simulink model "Noa_Nofusion_angle"  (R2020b)
settings: Solver=FixedStepDiscrete  StartTime=0.0  StopTime=Inf  FixedStep=0.01  RelTol=1e-3
PostLoadFcn:
  | if any(exist('dsrtsu_mdlpostloadfcn', 'file') ~= 0), dsrtsu_mdlpostloadfcn('Execute', bdroot); end
InitFcn:
  | , if any(exist('rtifpga_mdlclblib', 'file') ~= 0), rtifpga_mdlclblib('Init', bdroot); end,
  | , if any(exist('dsmpb_private', 'file') ~= 0), dsmpb_private('dsmpb_mdlclblib', 'Init', bdroot); end,
undefined symbols (not defined in the file): ACC_TimeGap_DecSetSwt, ACC_TimeGap_IncSetSwt, AccelPedalPosn, AccelPedalPosnVldty, AccelPedlPosnDiagc, AccPedalOverride, ACU_ShiftInProgress, ADAS_Posn_CurLane, AESSwtReq, ALC_SwtReq, BrkPedalSts, CC_ACC_CANCEL_OFFSwt, CC_ACC_CRUISE_OFFSwt, CC_ACC_DecSetSpd_SetSwt, CC_ACC_IncSetSpd_ResuSwt, CC_ACCSwtErr, CharSpd_ms, CSA_NODE, CURRENT_GEAR, CurrentGearValid, DiscIntNeverNeededParam, DrvDoorSts, DrvSBR, DrvTrqReqOvld, ECMACCInterface, ECMRespACC, ELKSwtReq, EngLimpHomeSts, EngSpd, EngState, EngState_PHEV, EngTrqMaxActSpd, EngTrqMinAct, EPS_DrvInpTrqVal_HighReslolution, EPS_FailSts, EPS_LKATorqOvrlDlvd, EPS_LKATorqOvrlDlvdVld, EPS_LKATrqOvlDlvdSts, EPS_SteerMod, EPS_TrqSnsrSts, EQ4_APPINFO, EQ4_LA_ELEM, EQ4_LA_HDR, EQ4_LAP_ELEM, EQ4_LAP_HDR, EQ4_LH_ELEM, EQ4_LH_HDR, EQ4_LRE_ELEM, EQ4_LRE_HDR, ESS_PedSwtReq, ESS_VehSwtReq, FFogLmpSts_F_Pbox, FLWheelDriveDirection, FLWheelSpd, FrntWiprSwtSts, FrntWshrSwtSts, FRWheelDriveDirection, FRWheelSpd, HazardLmpSwtSts, HCU_AccelPedalPosn_Diag ... (+151)
libraries: simulink x138, dsmpblib x33, canfdmsglib x10
(part 14 of 17)

== matlab function Noa_Nofusion_angle/TOS2/Subsystem1/ACCOSM/HWA_Task100ms1/Trajectory/Trajectory/AssignHighPriorityObjects ==
  data: ObjNumber input; TrajNumber input; BufNumber input; SlipDisLim input; ObjPrio input; ObjMatrix input; VxvRef input; ObjCntAlive input; ObjClass input; ObjDxv input; ObjDyv input; TrajUsedK1 input; TrajHistBufferBTrajEndK1 input; ObjTrajNumberK1 input; TrajCurrentIndexK1 input; TrajHistBufferBValidK1 input; TrajHistBufferDxvK1 input; TrajHistBufferDyvK1 input; TrajHistBufferTTimeStampK1 input; TrajHistBufferClassK1 input; TrajUsed output boolean; TrajHistBufferBTrajEnd output boolean; ObjTrajNumber output uint8; TrajCurrentIndex output uint8; TrajHistBufferBValid output boolean; TrajHistBufferDxv output single; TrajHistBufferDyv output single; TrajHistBufferTTimeStamp output single; TrajHistBufferClass output uint8
function [TrajUsed,TrajHistBufferBTrajEnd,ObjTrajNumber,TrajCurrentIndex,TrajHistBufferBValid,...
    TrajHistBufferDxv,TrajHistBufferDyv,...
    TrajHistBufferTTimeStamp,TrajHistBufferClass] = fcn(...
    ObjNumber,TrajNumber,BufNumber,SlipDisLim,ObjPrio,ObjMatrix,VxvRef,ObjCntAlive,ObjClass,ObjDxv,ObjDyv,...
    TrajUsedK1,TrajHistBufferBTrajEndK1,ObjTrajNumberK1,TrajCurrentIndexK1,...
    TrajHistBufferBValidK1,TrajHistBufferDxvK1,TrajHistBufferDyvK1,...
    TrajHistBufferTTimeStampK1,TrajHistBufferClassK1)

[TrajUsed,TrajHistBufferBTrajEnd,ObjTrajNumber,TrajCurrentIndex,TrajHistBufferBValid,...
    TrajHistBufferDxv,TrajHistBufferDyv,...
    TrajHistBufferTTimeStamp,TrajHistBufferClass] = Traj_AssignHighPriorityObjects(...
    ObjNumber,TrajNumber,BufNumber,SlipDisLim,ObjPrio,ObjMatrix,VxvRef,ObjCntAlive,ObjClass,ObjDxv,ObjDyv,...
    TrajUsedK1,TrajHistBufferBTrajEndK1,ObjTrajNumberK1,TrajCurrentIndexK1,...
    TrajHistBufferBValidK1,TrajHistBufferDxvK1,TrajHistBufferDyvK1,...
    TrajHistBufferTTimeStampK1,TrajHistBufferClassK1);
end

== matlab function Noa_Nofusion_angle/TOS2/Subsystem1/ACCOSM/HWA_Task100ms1/Trajectory/Trajectory/CalcCompensateEgoVehMove ==
  data: BufNumber input; TrajNumber input; tCycle input; dDeltaX input; dDeltaY input; CosOfPsi input; SinOfPsi input; TrajHistBufferBValidK1 input; TrajHistBufferDxvK1 input; TrajHistBufferDyvK1 input; TrajHistBufferBValid output; TrajHistBufferDxv output; TrajHistBufferDyv output; TrajHistBufferTTimeStampK1 input; TrajHistBufferTTimeStamp output
function [TrajHistBufferBValid,TrajHistBufferDxv,TrajHistBufferDyv,...
    TrajHistBufferTTimeStamp] = ...
    Compensate(BufNumber,TrajNumber,tCycle,dDeltaX,dDeltaY,CosOfPsi,SinOfPsi,...
    TrajHistBufferBValidK1,TrajHistBufferDxvK1,TrajHistBufferDyvK1,...
    TrajHistBufferTTimeStampK1)
%#codegen
TrajHistBufferBValid = TrajHistBufferBValidK1;
TrajHistBufferDxv = TrajHistBufferDxvK1;
TrajHistBufferDyv = TrajHistBufferDyvK1;
TrajHistBufferTTimeStamp = TrajHistBufferTTimeStampK1;

for i=1:TrajNumber
    for j=1:BufNumber
        if TrajHistBufferBValid(i,j)==true
            t_dx = TrajHistBufferDxv(i,j)-dDeltaX;
            t_dy = TrajHistBufferDyv(i,j)-dDeltaY;
            t_dxTmp = t_dx*CosOfPsi+t_dy*SinOfPsi;
            t_dyTmp = -t_dx*SinOfPsi+t_dy*CosOfPsi;
            if (t_dxTmp>-255)&&(t_dxTmp<255)&&(t_dyTmp>-255)&&(t_dyTmp<255)
                TrajHistBufferDxv(i,j) = t_dxTmp;
                TrajHistBufferDyv(i,j) = t_dyTmp;
            else
                TrajHistBufferBValid(i,j) = false;
            end
            
            TrajHistBufferTTimeStamp(i,j) = min(TrajHistBufferTTimeStamp(i,j)+tCycle,32);
            
            if TrajHistBufferDxv(i,j)<-1
                TrajHistBufferBValid(i,j) = false;
            end
        end
    end
end

== matlab function Noa_Nofusion_angle/TOS2/Subsystem1/ACCOSM/HWA_Task100ms1/Trajectory/Trajectory/CalcEgoVehMove ==
  data: dDeltaX output single size=1; tCycle input size=1; Kap input size=1; Vego input size=1; alpSideSlipAngle input size=1; dDeltaY output single size=1; CosOfPsi output single size=1; SinOfPsi output single size=1; WheelTrack input; SlipDislim output; Vch input
function [dDeltaX,dDeltaY,CosOfPsi,SinOfPsi,SlipDislim] = EgoVehicleMovement(tCycle,Kap,Vego,alpSideSlipAngle,WheelTrack,Vch)
%#codegen
if Kap==0
    dDeltaX = Vego*tCycle;
    dDeltaY = single(0);
    CosOfPsi = single(1);
    SinOfPsi = single(0);
    SlipDislim = Vch*1000;
else
    SlipDislim = max(WheelTrack*1000,min(tCycle*Vego,Kap*15));
    t_Psi = Kap*Vego*tCycle;
    SinOfPsi = sin(t_Psi);
    CosOfPsi = cos(t_Psi);
    t_dDeltaXTemp = SinOfPsi/Kap;
    t_dDeltaYTemp = 2*(sin(t_Psi/2)*sin(t_Psi/2))/Kap;
    dDeltaX = min(cos(alpSideSlipAngle)*t_dDeltaXTemp - sin(alpSideSlipAngle)*t_dDeltaYTemp,SlipDislim);
    dDeltaY = sin(alpSideSlipAngle)*t_dDeltaXTemp + cos(alpSideSlipAngle)*t_dDeltaYTemp;
end

== matlab function Noa_Nofusion_angle/TOS2/Subsystem1/ACCOSM/HWA_Task100ms1/Trajectory/Trajectory/Priority ==
  data: ObjNumber input; ObjValid input; ObjPrio output single; ObjClass input; ObjDx input; ObjMatrix output single
function [ObjPrio,ObjMatrix] = fcn(ObjNumber,ObjValid,ObjClass,ObjDx)
%#codegen
ObjPrio = single(zeros(15,1));

for i=1:ObjNumber
    if ObjValid(i)
        if ObjDx(i)<0
            ObjPrio(i)=single(0);
        else
            if (ObjClass(i)==2)||(ObjClass(i)==3)||(ObjClass(i)==5)
                t_ObjPrio=single(2*255);
            else
                t_ObjPrio=single(255);
            end
            ObjPrio(i) = t_ObjPrio - ObjDx(i);
        end
    else
        ObjPrio(i)=single(0);
    end
end

ObjMatrix=ObjPrio;

t_h=1;
while 1
    t_h = t_h*3+1;
    if t_h>=ObjNumber
        break;
    end
end

%   t_h = 121;
while 1
    t_h = fix(t_h/3);
    for i=(t_h+1):ObjNumber
        j=i;
        t_zw=ObjMatrix(i);
        while (j>t_h)&&(t_zw<ObjMatrix(j-t_h))
            ObjMatrix(j)=ObjMatrix(j-t_h);
            j=j-t_h;
        end
        ObjMatrix(j)=t_zw;
    end
    if t_h==1
        break;
    end
end

== matlab function Noa_Nofusion_angle/TOS2/Subsystem1/ACCOSM/HWA_Task100ms1/Trajectory/Trajectory/ReleaseLowPriorityObjects ==
  data: TrajUsed output; ObjNumber input; TrajNumber input; ObjPrio input; ObjMatrix input; ObjValid input; TrajCurrentIndex input; TrajUsedK1 input; TrajHistBufferBTrajEndK1 input; ObjTrajNumberK1 input; TrajHistBufferBTrajEnd output; ObjTrajNumber output
function [TrajUsed,TrajHistBufferBTrajEnd,ObjTrajNumber] =...
    fcn(ObjNumber,TrajNumber,ObjPrio,ObjMatrix,ObjValid,TrajCurrentIndex,...
    TrajUsedK1,TrajHistBufferBTrajEndK1,ObjTrajNumberK1)
%#codegen
TrajHistBufferBTrajEnd = TrajHistBufferBTrajEndK1;
TrajUsed = TrajUsedK1;
ObjTrajNumber = ObjTrajNumberK1;
ObjPrioLimit = ObjMatrix(ObjNumber-TrajNumber);

for i=1:ObjNumber
    if ObjValid(i)
        if (ObjPrio(i)==0)||(ObjPrio(i)<=ObjPrioLimit)
            j = ObjTrajNumber(i);
            if j<(TrajNumber+1)
                t = TrajCurrentIndex(j);
                TrajHistBufferBTrajEnd(j,t)=1;
                TrajUsed(j)=0;
                ObjTrajNumber(i)=255;
            end
        end
    end
end

== matlab function Noa_Nofusion_angle/TOS2/Subsystem1/ACCOSM/HWA_Task100ms1/Trajectory/Trajectory/StoreEgoTrajectory ==
  data: Pa output single; Pb output single; Pc output single; Pd output single; BufNumber input; tCycle input; EgoTrajHistCurrentIndex output uint8; EgoDDeltaX input; EgoDDeltaY input; EgoCosOfPsi input; EgoSinOfPsi input; EgoTrajHistDxv output; EgoTrajHistDyv output; EgoTrajHistTTimeStamp output; EgoTrajHistCurrentIndexK1 input; EgoTrajHistDxvK1 input single; EgoTrajHistDyvK1 input single; EgoTrajHistTTimeStampK1 input single
function [Pa,Pb,Pc,Pd,EgoTrajHistCurrentIndex,EgoTrajHistDxv,EgoTrajHistDyv,EgoTrajHistTTimeStamp]...
    = fcn(BufNumber,tCycle,EgoDDeltaX,EgoDDeltaY,EgoCosOfPsi,EgoSinOfPsi,...
    EgoTrajHistCurrentIndexK1,EgoTrajHistDxvK1,EgoTrajHistDyvK1,EgoTrajHistTTimeStampK1)
%#codegen
EgoTrajHistCurrentIndex = EgoTrajHistCurrentIndexK1;
EgoTrajHistDxv = EgoTrajHistDxvK1;
EgoTrajHistDyv = EgoTrajHistDyvK1;
EgoTrajHistTTimeStamp = EgoTrajHistTTimeStampK1;
% alpWheelAngleOffset = alpWheelAngleOffsetK1;

t_IdxActualElement = EgoTrajHistCurrentIndex;
if t_IdxActualElement==BufNumber
    t_IdxNextElement=uint8(1);
else
    t_IdxNextElement=t_IdxActualElement+1;
end

Temp1 = EgoTrajHistDxv(t_IdxActualElement) - EgoDDeltaX;
Temp2 = EgoTrajHistDyv(t_IdxActualElement) - EgoDDeltaY;
dDeltaS = Temp1*Temp1 + Temp2*Temp2;
t_AddPosition = ((EgoTrajHistTTimeStamp(t_IdxActualElement)+tCycle)>0.3);
t_AddPosition = t_AddPosition&(dDeltaS>4);
t_AddPosition = t_AddPosition|(dDeltaS>100);
for iBuf=1:BufNumber
    if (t_AddPosition==1)&&(iBuf==t_IdxNextElement)
        EgoTrajHistDxv(iBuf)=single(0);
        EgoTrajHistDyv(iBuf)=single(0);
        EgoTrajHistTTimeStamp(iBuf)=single(0);
        EgoTrajHistCurrentIndex = t_IdxNextElement;
    else
        dX = EgoTrajHistDxv(iBuf)-EgoDDeltaX;
        dY = EgoTrajHistDyv(iBuf)-EgoDDeltaY;
        if (EgoTrajHistDxv(iBuf)>-255)&&(dX>-255)&&(dX<255)&&(dY>-255)&&(dY<255)
            Temp1 = dX*EgoCosOfPsi + dY*EgoSinOfPsi;
            Temp2 = -dX*EgoSinOfPsi + dY*EgoCosOfPsi;
            if (Temp1>-255)&&(Temp1<255)&&(Temp2>-255)&&(Temp2<255)
                EgoTrajHistDxv(iBuf)=Temp1;
                EgoTrajHistDyv(iBuf)=Temp2;
                tDt = EgoTrajHistTTimeStamp(iBuf)+tCycle;
                if tDt>32
                    tDt=single(32);
                end
                EgoTrajHistTTimeStamp(iBuf) = tDt;
            else
                EgoTrajHistDxv(iBuf)=single(-255);
                EgoTrajHistDyv(iBuf)=single(-255);
                EgoTrajHistTTimeStamp(iBuf) = single(32);
            end
        else
            EgoTrajHistDxv(iBuf)=single(-255);
            EgoTrajHistDyv(iBuf)=single(-255);
            EgoTrajHistTTimeStamp(iBuf) = single(32);
        end
    end
end

t_Index = EgoTrajHistCurrentIndex;
t_Index1 = BufNumber + uint8(23);
t_Index2 = BufNumber + uint8(21);
t_Index3 = BufNumber + uint8(19);

if t_Index1>24
    t_Index1 = t_Index1 - uint8(24);
end
if t_Index2>24
    t_Index2 = t_Index2 - uint8(24);
end
if t_Index3>24
    t_Index3 = t_Index3 - uint8(24);
end

XiMa = [EgoTrajHistDxv(t_Index);EgoTrajHistDxv(t_Index1);EgoTrajHistDxv(t_Index2);EgoTrajHistDxv(t_Index3)];
YiMa = [EgoTrajHistDyv(t_Index);EgoTrajHistDyv(t_Index1);EgoTrajHistDyv(t_Index2);EgoTrajHistDyv(t_Index3)];

[Pa,Pb,Pc,Pd] = pl(XiMa,YiMa);

% if (abs(EgoTrajHistDyv(t_Index1))<0.1)&&(abs(EgoTrajHistDyv(t_Index2))<0.1)&&(abs(EgoTrajHistDyv(t_Index3))<0.1)
%     kapRef = 3*Pa*EgoTrajHistDxv(t_Index2) + 2*Pb;
%     AckConst = min((1+VxvRef*VxvRef/(26*26))*2.68/max(VxvRef,1),32767);
%     alpWheelAngleRef = VxvRef*kapRef*AckConst;
%     Raw = alpWheelAngleMean - alpWheelAngleRef;
%     if VxvRef>7.3
%         alpWheelAngleOffset = (Raw - alpWheelAngleOffset)/10000 + alpWheelAngleOffset;
%     end
% else
%     alpWheelAngleRef = single(255);
% end

== matlab function Noa_Nofusion_angle/TOS2/Subsystem1/ACCOSM/HWA_Task100ms1/VycCalc ==
  data: ObjVyc output single size=15; dxC0 input; aP0 input; bP0 input; aP1 input; bP1 input; ObjValid input boolean size=15; ObjDx input single size=15; ObjVxG input single size=15; ObjVyG input single size=15; ObjYawAngle output
function [ObjVyc,ObjYawAngle] = VycCalc(dxC0,aP0,bP0,aP1,bP1,ObjValid,ObjDx,ObjVxG,ObjVyG)

ObjVyc = single(zeros(15,1));
ObjYawAngle = single(zeros(15,1));

for i=1:15
    if ObjValid(i)
       t_dxv = ObjDx(i);
       t_VxG = ObjVxG(i);
       t_VyG = ObjVyG(i);
       
       if abs(t_VxG)<0.1
          if t_VyG>0.5
              ObjYawAngle(i) = single(1.57);
          end
          if t_VyG<-0.5
              ObjYawAngle(i) = single(-1.57);
          end
       else
           if t_VxG>0
               ObjYawAngle(i) = atan(t_VyG/t_VxG);
           else
               if t_VyG>0
                  ObjYawAngle(i) = single(3.1416) + atan(t_VyG/t_VxG);
               else
                  ObjYawAngle(i) = -single(3.1416) + atan(t_VyG/t_VxG);
               end
           end
       end
       
       t_bParabolaYNLane = single(1);
       if t_dxv<dxC0
          temp1 =  2*aP0*t_dxv + bP0;
          t_bParabolaXNLane = -temp1;
       else
          temp1 =  2*aP1*t_dxv + bP1;
          t_bParabolaXNLane = -temp1;
       end
       t_bParabolaMag = mag(t_bParabolaXNLane,t_bParabolaYNLane);
       t_bParabolaXNLane = t_bParabolaXNLane/t_bParabolaMag;
       t_bParabolaYNLane = t_bParabolaYNLane/t_bParabolaMag;
       temp1 = t_VxG*t_bParabolaXNLane;
       temp2 = t_VyG*t_bParabolaYNLane;
       
       ObjVyc(i) = temp1 + temp2;
    else
       ObjVyc(i) = single(0);
    end
end
end

function out = mag(x,y)
M = max(abs(x),abs(y));
N = min(abs(x),abs(y));
out = M + 0.322*N;
end

== matlab function Noa_Nofusion_angle/TOS2/Subsystem1/ACCOSM/HWA_Task100ms1/dyLaneWidthSteerAdapt ==
  data: kap input; dyLaneAdaptLeft output; dyAdapt input; dyLaneAdaptRight output
function [dyLaneAdaptLeft,dyLaneAdaptRight] = fcn(kap,dyAdapt)

dyLaneAdaptLeft = single(0);
dyLaneAdaptRight = single(0);
if kap>0
    dyLaneAdaptRight = dyAdapt;
end
if kap<0
    dyLaneAdaptLeft = dyAdapt;
end

== matlab function Noa_Nofusion_angle/TOS2/Subsystem1/ACCOSM/HWA_Task100ms1/wCutInVy ==
  data: DycASI output single; ObjValid input boolean size=15; ObjDycCutIn input single size=15; ObjWidth input single size=15; ObjVyc input single size=15; ObjDx input single size=15; ObjDy input single size=15; ObjCnt input uint8 size=15; ObjDycFilt input single size=15; ObjwCutInVyK1 input single size=15; ObjtPrediction4CutIn output single size=15; ObjDycCutInPredict output single size=15; ObjCutIn_b output boolean size=15; ObjwCutInVy output single size=15
function [DycASI,ObjtPrediction4CutIn,ObjDycCutInPredict,ObjCutIn_b,ObjwCutInVy] = ...
    CalcWCutInVy(ObjValid,ObjDycCutIn,ObjWidth,ObjVyc,ObjDx,ObjDy,ObjCnt,...
    ObjDycFilt,ObjwCutInVyK1)
 
ObjwCutInVy = single(zeros(15,1));
ObjtPrediction4CutIn = single(zeros(15,1));
ObjDycCutInPredict = single(zeros(15,1));
DycASI = single(zeros(15,1));
ObjCutIn_b = false(15,1);
 
for i=1:15
    if ObjValid(i)
        dWidth = ObjWidth(i);
        dycASI = ObjDycCutIn(i);
        vyc = ObjVyc(i);
        dx = ObjDx(i);
        dy = ObjDy(i);
        dycFilt = ObjDycFilt(i);
        wCutInVyK1 = ObjwCutInVyK1(i);
  
        temp1 = dycFilt - dycASI;
        if ((dycASI>0)&&(temp1>0.2))||((dycASI<0)&&(temp1<-0.2))
            tauVy = single(1.6);
        else
            tauVy = single(0);
        end
        tauVy = interpolate(single(40),tauVy,single(70),single(0),dx);
        ObjtPrediction4CutIn(i) = tauVy;
        temp1 = vyc*tauVy;
        temp2 = dycASI + temp1;
        
        if (dycASI>0)&&(temp2<0)
            temp2 = single(0);
        else
            if (dycASI<0)&&(temp2>0)
                temp2 = single(0);
            else
                if dycASI==0
                    temp2 = single(0);
                end
            end
        end
        ObjDycCutInPredict(i) = temp2;
        if dycASI>0
            temp1 = temp2 - 0.5*dWidth;
            t_dycASI = max(temp1,single(0));
        else
            temp1 = temp2 + 0.5*dWidth;
            t_dycASI = min(temp1,single(0));
        end
        temp1 = abs(t_dycASI);
        t_wCutInVy = interpolate(single(0),single(1),single(0.7),single(0),temp1);
        if tauVy==0
            t_wCutInVy = single(0);
        end
        
        if dx>0
            fak = abs(dy)/dx; 
        else
            fak = single(0);
        end
        if (ObjCnt(i)<2)||(abs(dy)>=2.4)||(fak>0.25)
           t_wCutInVy = single(0);
        end
       
        temp1 = t_wCutInVy - wCutInVyK1;
        temp1_ub = abs(temp1);
        temp2 = 0.2*temp1_ub;
        if temp1>0
            t_wCutInVy = wCutInVyK1 + temp2;
        else
            t_wCutInVy = wCutInVyK1 - temp2;
        end
        ObjwCutInVy(i) = t_wCutInVy;
        DycASI(i) = t_dycASI;
        if t_wCutInVy>0.7
            ObjCutIn_b(i) = true;
        end
    end
end
end
 
% function out = interpolate(x1,z1,x2,z2,Raw)
% if Raw<=x1
%     out = z1;
% else
%     if Raw>=x2
%         out = z2;
%     else
%         out = z1 + (Raw-x1)*(z2-z1)/(x2-x1);
%     end
% end
% end

== matlab function Noa_Nofusion_angle/TOS2/Subsystem1/ACCOSM/HWA_Task100ms1/wCutOutVy ==
  data: vRef input single size=1; kap input single size=1; tDirIndLeft input single size=1; tDirIndRight input single size=1; ObjValid input boolean size=15; ObjDycCutIn input single size=15; ObjWidth input single size=15; ObjtPrediction4CutOut output single size=15; ObjDycCutOutPredict output single size=15; ObjwCutOutTurnOff output single size=15; ObjVyc input single size=15; ObjDx input single size=15; ObjDy input single size=15; ObjVx input single size=15; ObjVy input single size=15; ObjDyc input single size=15; ObjDrive_b input boolean size=15; ObjCnt input uint8 size=15; ObjDycFilt input single size=15; ObjwCutoutVyK1 input single size=15; ObjwCutoutVy output single size=15
function [ObjtPrediction4CutOut,ObjDycCutOutPredict,ObjwCutOutTurnOff,ObjwCutoutVy] = ...
    CalcWCutOutVy(vRef,kap,tDirIndLeft,tDirIndRight,ObjValid,ObjDycCutIn,ObjWidth,...
    ObjVyc,ObjDx,ObjDy,ObjVx,ObjVy,ObjDyc,ObjDrive_b,ObjCnt,...
    ObjDycFilt,ObjwCutoutVyK1)
 
ObjwCutoutVy = single(zeros(15,1));
ObjtPrediction4CutOut = single(zeros(15,1));
ObjDycCutOutPredict = single(zeros(15,1));
ObjwCutOutTurnOff = single(zeros(15,1));
 
for i=1:15
    if ObjValid(i)
        dWidth = ObjWidth(i);
        dycASI = ObjDycCutIn(i);
        vyc = ObjVyc(i);
        dx = ObjDx(i);
        dy = ObjDy(i);
        vx = ObjVx(i);
        vy = ObjVy(i);
        dyc = ObjDyc(i);
        dycFilt = ObjDycFilt(i);
        wCutoutVyK1 = ObjwCutoutVyK1(i);
        Move_b = ObjDrive_b(i);
        Cnt = ObjCnt(i);
        t_vxTO = vRef + vx;
        t_vxvThreshold = 0.5 - vRef;
        
        temp1 = dycASI - dycFilt;
        if ((dycASI>0)&&(temp1>0.2))||((dycASI<0)&&(temp1<-0.2))
            tauVy = single(1);
        else
            tauVy = single(0);
        end
        tauVy = interpolate(single(40),tauVy,single(70),single(0),dx);
        ObjtPrediction4CutOut(i) = tauVy;
        temp1 = vyc*tauVy;
        temp2 = dycASI + temp1;
        
        if (dycASI>0)&&(temp2<0)
            temp2 = single(0);
        else
            if (dycASI<0)&&(temp2>0)
                temp2 = single(0);
            else
                if dycASI==0
                    temp2 = single(0);
                end
            end
        end
        ObjDycCutOutPredict(i) = temp2;
        if dycASI>0
            temp1 = temp2 + 0.5*dWidth;
            t_dycASI = max(temp1,single(0));
        else
            temp1 = temp2 - 0.5*dWidth;
            t_dycASI = min(temp1,single(0));
        end
        temp1 = abs(t_dycASI);
        t_wCutoutVy = interpolate(single(0),single(0),single(0.7),single(1),temp1);
        if tauVy==0
            t_wCutoutVy = single(0);
        end
        
        temp1 = t_wCutoutVy - wCutoutVyK1;
        temp1_ub = abs(temp1);
        temp2 = 0.2*temp1_ub;
        if temp1>0
            t_wCutoutVy = wCutoutVyK1 + temp2;
        else
            t_wCutoutVy = wCutoutVyK1 - temp2;
        end
        ObjwCutoutVy(i) = t_wCutoutVy;
        if (dx<30)&&(Move_b==true)&&(vRef>0.5)&&(t_vxTO<6)&&(vx>t_vxvThreshold)&&(abs(dyc)>0.5)&&...
        (abs(dy)>0.5)&&(abs(dy)<4)&&(abs(vy)>0.5)&&...
        (((dyc<0)&&(vyc<0)&&(tDirIndRight==0))||((dyc>0)&&(vyc>0)&&(tDirIndLeft==0)))&&...
        (kap>-0.005)&&(kap<0.005)&&...
        (Cnt==7) 
             ObjwCutOutTurnOff(i) = t_wCutoutVy;
        end
    end
end
end

== matlab function Noa_Nofusion_angle/TOS2/Subsystem1/ACCOSM/ObjMatrixTransit/Subsystem/MATLAB Function1 ==
  data: P output uint8; Count input uint8 size=1; ID input uint8 size=20; BrakeLight_b input uint8 size=20; Class input uint8 size=20; LatDis input single size=20; LatVel input single size=20; LongAccel input single size=20; LongDis input single size=20; LongVel input single size=20; Width input single size=20; Age input uint16 size=20; MotionSts input uint8 size=20; ObjValid output boolean size=20; ObjBrakeLightIndic output uint8 size=20; ObjClassification output uint8 size=20; ObjLatPos output single size=20; ObjLatVel output single size=20; ObjLongAccel output single size=20; ObjLongVel output single size=20; ObjWidth output single size=20; ObjCnt output uint8 size=20; ObjMoveSts output uint8 size=20; ObjLongPos output single size=20; ObjIDK1 input uint8 size=20; ObjID output uint8 size=20
function [P,ObjValid,ObjBrakeLightIndic,ObjClassification,...
    ObjLatPos,ObjLatVel,ObjLongAccel,ObjLongVel,...
    ObjWidth,ObjCnt,ObjMoveSts,ObjLongPos,ObjID] =...
    DataT(Count,ID,BrakeLight_b,Class,LatDis,LatVel,LongAccel,LongDis,LongVel,Width,Age,MotionSts,ObjIDK1)

ObjValid = false(20,1);
ObjID = uint8(zeros(20,1));
ObjBrakeLightIndic = uint8(zeros(20,1));
ObjClassification = uint8(zeros(20,1));
ObjLatPos = single(zeros(20,1));
ObjLatVel = single(zeros(20,1));
ObjLongAccel = single(zeros(20,1));
ObjLongPos = single(zeros(20,1));
ObjLongVel = single(zeros(20,1));
ObjWidth = single(zeros(20,1));
ObjCnt = uint8(zeros(20,1));
ObjMoveSts = uint8(zeros(20,1));

T = uint8(zeros(20,1));
P = uint8(zeros(20,1));
Index01 = uint8(zeros(20,1));
Index02 = uint8(zeros(20,1));
M = uint8(0);
N = uint8(0);
w = uint8(0);

for i=uint8(1):Count
    for j=uint8(1):uint8(20)
        if ID(i)==ObjIDK1(j)
            T(j) = i;
            P(i) = j;
        end
    end
end

for j=uint8(1):uint8(20)
    if T(j)==uint8(0)
        if ObjIDK1(j)==uint8(0)
            N = N + uint8(1);
            Index01(N) = j;
        else
            M = M + uint8(1);
            Index02(M) = j;
        end
        ObjValid(j) = false;
    else
        ObjValid(j) = true;
    end
end

for i=uint8(1):Count
    if P(i)==uint8(0)
        w = w + uint8(1);
        if w<=N
            P(i) = Index01(w);
        else
            P(i) = Index02(w - N);
        end
        ObjValid(Index01(w)) = true;
    end
    ObjID(P(i)) = ID(i);
    if BrakeLight_b(i)==uint8(1)
        ObjBrakeLightIndic(P(i)) = uint8(2);
    end
    if Class(i)==uint8(1)||Class(i)==uint8(2)||...
            Class(i)==uint8(3)||Class(i)==uint8(6)
        ObjClassification(P(i)) = uint8(1);
    end
    ObjLatPos(P(i)) = -LatDis(i) - single(0.1);
    ObjLatVel(P(i)) = -LatVel(i);
    ObjLongAccel(P(i)) = LongAccel(i);
    ObjLongPos(P(i)) = LongDis(i);
    ObjLongVel(P(i)) = LongVel(i);
    ObjWidth(P(i)) = Width(i);
    if Age(i)<=255
        ObjCnt(P(i)) = uint8(Age(i)/2) - uint8(1);
    else
        ObjCnt(P(i)) = uint8(127);
    end
    if MotionSts(i)==uint8(1)||MotionSts(i)==uint8(3)
        ObjMoveSts(P(i)) = uint8(1);
    elseif MotionSts(i)==uint8(2)||MotionSts(i)==uint8(5)
        if LongVel(i)>-2.5
            ObjMoveSts(P(i)) = uint8(2);
        else
            ObjMoveSts(P(i)) = uint8(4);
        end
    elseif MotionSts(i)==uint8(4)
        ObjMoveSts(P(i)) = uint8(3);
    end
end
end

== stateflow chart Noa_Nofusion_angle/TOS2/Subsystem1/ACCOSM/ObjMatrixTransit/Subsystem/Obj ==
  (default) -> (junction 5)
  (junction 5) -> (junction 36) : {i=1;}
  (junction 36) -> (junction 38) [order 1] : [i<21]
  (junction 40) -> (junction 36) : {i=i+1;}
  (junction 36) -> (junction 42) [order 2]
  (junction 38) -> (junction 40) : {id(i) = IFV410_Obj(i).OBJ_ID;
      | confidence(i) = IFV410_Obj(i).OBJ_Existence_Probability;
      | classification(i) = IFV410_Obj(i).OBJ_Object_Class;
      | width(i) = IFV410_Obj(i).OBJ_Width;
      | LongDis(i) = IFV410_Obj(i).OBJ_Long_Distance;
      | LatDis(i) = IFV410_Obj(i).OBJ_Lat_Distance;
      | AbsLongAcc(i) = IFV410_Obj(i).OBJ_Abs_Long_Acc;
      | AbsLongVel(i) = IFV410_Obj(i).OBJ_Abs_Long_Velocity;
      | AbsLatVel(i) = IFV410_Obj(i).OBJ_Abs_Lat_Velocity;
      | BrakeLight(i) = IFV410_Obj(i).OBJ_Brake_Light;
      | Age(i) = IFV410_Obj(i).OBJ_Object_Age;
      | motionSts(i) = IFV410_Obj(i).OBJ_Motion_Status;
      | motionCategory(i) = IFV410_Obj(i).OBJ_Motion_Category;
      | motionOrientation(i) = IFV410_Obj(i).OBJ_Motion_Orientation;}
  data: i local uint8; id output uint8 size=20 =uint8(zeros(20,1)); classification output uint8 size=20 =uint8(zeros(20,1)); AbsLongAcc output single size=20 =single(zeros(20,1)); width output single size=20 =single(zeros(20,1)); AbsLongVel output single size=20 =single(zeros(20,1)); LongDis output single size=20 =single(zeros(20,1)); AbsLatVel output single size=20 =single(zeros(20,1)); LatDis output single size=20 =single(zeros(20,1)); BrakeLight output uint8 size=20 =uint8(zeros(20,1)); Age output uint16 size=20 =uint16(zeros(20,1)); confidence output single size=20 =single(zeros(20,1)); IFV410_Obj input Bus: SPI_EQ4_OBJ_ELEM_BUS size=20; motionSts output uint8 size=20 =uint8(zeros(20,1)); motionCategory output uint8 size=20 =uint8(zeros(20,1)); motionOrientation output uint8 size=20 =uint8(zeros(20,1))

== matlab function Noa_Nofusion_angle/TOS/Subsystem1/ACCOSM/HWA_Task100ms1/ACC_DisplayBar ==
  data: TimeGap input; DisplayBar output uint8; DesireDistance input; ACCmode input; TargetRange input; Scale input; TargetExist input; DisplayBarK1 input uint8
function DisplayBar = fcn(TimeGap,DesireDistance,ACCmode,TargetRange,Scale,TargetExist,DisplayBarK1)
%#codegen
DisplayBar = DisplayBarK1;

ScaleDis = Scale*DesireDistance;
upScaleDis = (Scale+single(0.05))*DesireDistance;
lowScaleDis = (Scale-single(0.05))*DesireDistance;

i = TimeGap;

if (ACCmode==0)||(ACCmode==7)
    DisplayBar = uint8(0);
else
    if TargetExist==false
        DisplayBar=uint8(0);
    else
        switch(DisplayBarK1)
            case uint8(0)
                 if TargetRange> ScaleDis(i,3)
                     DisplayBar=uint8(4);
                 else
                     if TargetRange>ScaleDis(i,2)
                         DisplayBar=uint8(3);
                     else
                         if TargetRange>ScaleDis(i,1)
                             DisplayBar=uint8(2);
                         else
                             DisplayBar=uint8(1);
                         end
                     end
                 end
            case uint8(1)
                 if TargetRange> upScaleDis(i,3)
                     DisplayBar=uint8(4);
                 else
                     if TargetRange>upScaleDis(i,2)
                         DisplayBar=uint8(3);
                     else
                         if TargetRange>upScaleDis(i,1)
                             DisplayBar=uint8(2);
                         else
                             DisplayBar=uint8(1);
                         end
                     end
                 end
            case uint8(2)
                 if TargetRange> upScaleDis(i,3)
                     DisplayBar=uint8(4);
                 else
                     if TargetRange>upScaleDis(i,2)
                         DisplayBar=uint8(3);
                     else
                         if TargetRange>lowScaleDis(i,1)
                             DisplayBar=uint8(2);
                         else
                             DisplayBar=uint8(1);
                         end
                     end
                 end   
            case uint8(3)
                 if TargetRange> upScaleDis(i,3)
                     DisplayBar=uint8(4);
                 else
                     if TargetRange>lowScaleDis(i,2)
                         DisplayBar=uint8(3);
                     else
                         if TargetRange>lowScaleDis(i,1)
                             DisplayBar=uint8(2);
                         else
                             DisplayBar=uint8(1);
                         end
                     end
                end
            case uint8(4)
                 if TargetRange> lowScaleDis(i,3)
                     DisplayBar=uint8(4);
                 else
                     if TargetRange>lowScaleDis(i,2)
                         DisplayBar=uint8(3);
                     else
                         if TargetRange>lowScaleDis(i,1)
                             DisplayBar=uint8(2);
                         else
                             DisplayBar=uint8(1);
                         end
                     end
                 end      
        end    
    end
end

== matlab function Noa_Nofusion_angle/TOS/Subsystem1/ACCOSM/HWA_Task100ms1/Dyc ==
  data: kapTrajFiltK1 input single size=1; vRef input single size=1; kapTrajFilt output single size=1; kapCourseErr output single; kapTraj input single size=1; alpSideSlipAngle input single size=1; A2 input single size=1; A1 input single size=1; LineValid input boolean size=1; ObjDx input single size=15; ObjDy input single size=15; TarLineValid input boolean; TarLineA2 input single; TarLineA1 input single; TarLineA0 input single size=1; dxC0 output single size=1; aPC0 output single size=1; bPC0 output single size=1; cPC0 output single size=1; aPC1 output single size=1; bPC1 output single size=1; cPC1 output single size=1; ObjDyc output single size=15
function [kapTrajFilt,kapCourseErr,dxC0,aPC0,bPC0,cPC0,aPC1,bPC1,cPC1,ObjDyc] = ...
    DriveCourseCalc(kapTrajFiltK1,vRef,kapTraj,alpSideSlipAngle,...
    A2,A1,LineValid,ObjDx,ObjDy,TarLineValid,TarLineA2,TarLineA1,TarLineA0)

ObjDyc = single(zeros(15,1));

if vRef>8.33
    t_alpSideSlipAngle = -alpSideSlipAngle;
else
    t_alpSideSlipAngle = single(0);
end

temp1 = single(0.1)/(single(0.1) + interpolate(single(24),single(0),single(55),single(0.4),vRef));

kapTrajFilt = kapTrajFiltK1 + temp1*(kapTraj - kapTrajFiltK1);

temp1 = abs(kapTraj*vRef);

if (temp1<0.001)&&(vRef>8.3)
    t_kapTrajwHyst = single(0);
else
    t_kapTrajwHyst = kapTrajFilt;
end

if TarLineValid
    temp = interpolate(single(0.2),single(0.2),single(1.5),single(1),abs(TarLineA0));
    dxC0Min = single(3);
else
    temp = single(1);
    dxC0Min = single(10);
end

dxC0 = max(vRef*temp,dxC0Min);
aPC0 = 0.5*t_kapTrajwHyst*(single(1)+1.5*t_alpSideSlipAngle*t_alpSideSlipAngle);
bPC0 = t_alpSideSlipAngle;
cPC0 = single(0);

temp1 = single(0.1)*abs(t_kapTrajwHyst);
temp2 = min(single(0.00013),single(0.004)/max(vRef,single(10)));
kapCourseErr = max(temp1,temp2);

aPC1 = aPC0;
bPC1 = bPC0;
cPC1 = single(0);

Low = interpolate(single(4),single(1),single(20),single(0),abs(atan(A1)));    % low vehiclespeed lanechange Angle is 4deg~20deg;
High = interpolate(single(4),single(1),single(10),single(0),abs(atan(A1)));   % low vehiclespeed lanechange Angle is 4deg~10deg;
t_vRefFactor = interpolate(single(5),Low,single(25),High,vRef);

t_Factor = single(1)*t_vRefFactor;

if TarLineValid==true
    aPC1 = TarLineA2;
    bPC1 = TarLineA1;
    cPC1 = (aPC0 - aPC1)*dxC0*dxC0 + (bPC0 - bPC1)*dxC0;
else
    if LineValid
        aPC1 = aPC0*(1 - t_Factor) + A2*t_Factor;
        bPC1 = bPC0*(1 - t_Factor) + A1*t_Factor;
        cPC1 = (aPC0 - aPC1)*dxC0*dxC0 + (bPC0 - bPC1)*dxC0;
    end
end

for i=1:15
   if ObjDx(i)>dxC0
      ObjDyc(i) =  ObjDy(i) - (aPC1*ObjDx(i)*ObjDx(i) + bPC1*ObjDx(i) + cPC1);
   else
      ObjDyc(i) =  ObjDy(i) - (aPC0*ObjDx(i)*ObjDx(i) + bPC0*ObjDx(i));
   end
end
end


function out = interpolate(x1,z1,x2,z2,Raw)
if Raw<=x1
    out = z1;
else
    if Raw>=x2
        out = z2;
    else
        out = z1 + (Raw-x1)*(z2-z1)/(x2-x1);
    end
end
end

== matlab function Noa_Nofusion_angle/TOS/Subsystem1/ACCOSM/HWA_Task100ms1/DycCutIn ==
  data: ObjValid input boolean size=15; ObjDyc input single size=15; ObjMoveSts input uint8 size=15; ObjDycCutIn output single size=15; ObjMove_b output boolean size=15; ObjCnt input uint8 size=15; ObjDycHist input single size=15; ObjqDycHist input single size=15; dycFiltK1 input single size=15; ObjDycFilt output single size=15
function [ObjDycCutIn,ObjMove_b,ObjDycFilt] = ...
    ObjDycCutInCalc(ObjValid,ObjDyc,ObjMoveSts,ObjCnt,ObjDycHist,ObjqDycHist,dycFiltK1)
 
ObjDycCutIn = single(zeros(15,1));
ObjDycFilt = single(zeros(15,1));
ObjMove_b = false(15,1); 
 
for i=1:15
    if ObjValid(i)
        t_dyc = ObjDyc(i);
        t_dycHist = ObjDycHist(i);
        t_qDycHist = ObjqDycHist(i);
        
        weightDycHist = t_qDycHist*0.1;
        weightDyc = single(1) - weightDycHist;
        
        t_dycASI = weightDycHist*t_dycHist + weightDyc*t_dyc;
        ObjDycCutIn(i) = t_dycASI;
        
        if ObjCnt(i)>2
            ObjDycFilt(i) = 0.028*(t_dycASI - dycFiltK1(i)) + dycFiltK1(i);
        else
            ObjDycFilt(i) = t_dycASI;
        end
        if ObjMoveSts(i)==2
            ObjMove_b(i) = true;
        end
    end
end

== matlab function Noa_Nofusion_angle/TOS/Subsystem1/ACCOSM/HWA_Task100ms1/DycHistCalc ==
  data: TrajHistBufferBTrajEnd input boolean; ObjTrajNumber input uint8; ObjDycHist output single; TrajCurrentIndex input uint8; TrajHistBufferBValid input boolean; TrajHistBufferDxv input single; TrajHistBufferDyv input single; ObjValid input boolean; ObjqDycHist output single; dxC0 input; aP0 input; bP0 input; cP0 input; aP1 input; bP1 input; cP1 input
function [ObjDycHist,ObjqDycHist] = DycHistCalc(TrajHistBufferBTrajEnd,ObjTrajNumber,TrajCurrentIndex,...
    TrajHistBufferBValid,TrajHistBufferDxv,TrajHistBufferDyv,ObjValid,dxC0,aP0,bP0,cP0,aP1,bP1,cP1)

t_dxv = single(0);
t_dyv = single(0);
t_dxvK1 = single(0);
t_dyvK1 = single(0);
ObjDycHist = single(zeros(15,1));
ObjqDycHist = single(zeros(15,1));

for iObj=1:15
    t_TrajNumber = ObjTrajNumber(iObj);
    if t_TrajNumber<21
        t_End = false;
        t_Failed = false;
        t_TrajCurrentIndex = TrajCurrentIndex(t_TrajNumber);
        t_TrajEnd = TrajHistBufferBTrajEnd(t_TrajNumber,t_TrajCurrentIndex);
        if (ObjValid(iObj)==true)&&(t_TrajEnd==false)
            for k=1:24
                if t_End==false
                    if t_TrajCurrentIndex<k
                        t_Index = t_TrajCurrentIndex + uint8(25) - k;
                    else
                        t_Index = t_TrajCurrentIndex - k + uint8(1);
                    end
                    if t_Index==1
                        t_IndexK1 = uint8(24);
                    else
                        t_IndexK1 = t_Index - uint8(1);
                    end
                    t_ValidK1 = TrajHistBufferBValid(t_TrajNumber,t_IndexK1);
                    t_TrajEndK1 = TrajHistBufferBTrajEnd(t_TrajNumber,t_IndexK1);
                    t_dxv = TrajHistBufferDxv(t_TrajNumber,t_Index);
                    t_dxvK1 = TrajHistBufferDxv(t_TrajNumber,t_IndexK1);
                    t_dyv = TrajHistBufferDyv(t_TrajNumber,t_Index);
                    t_dyvK1 = TrajHistBufferDyv(t_TrajNumber,t_IndexK1);
                    
                    if (t_TrajEndK1==true)||(t_ValidK1==false)
                        t_End = true;
                        t_Failed = true;
                    end
                    if (t_dxv>=0)&&(t_dxvK1<=0)
                        t_End = true;
                    end
                end
            end
        end
        if (t_End==true)&&(t_Failed==false)
            if (t_dxv==t_dxvK1)
                t_dycHist = t_dyv;
            else
                t_dycHist = t_dyv - t_dxv*(t_dyvK1 - t_dyv)/(t_dxvK1 - t_dxv);
            end
            t_qDycHist = single(1);  
        else
            if (t_End==true)&&(t_Failed==true)&&(t_dxv>0)
                if t_dxv>(dxC0)
                    t_dycHist = t_dyv - (aP1*t_dxv*t_dxv + bP1*t_dxv + cP1); 
                else
                    t_dycHist = t_dyv - (aP0*t_dxv*t_dxv + bP0*t_dxv + cP0); 
                end
               t_qDycHist = max((single(80) - t_dxv)/single(80),single(0));
            else
                t_dycHist = single(0);
                t_qDycHist = single(0);
            end
        end
    else
        t_dycHist = single(0);
        t_qDycHist = single(0);
    end
    ObjDycHist(iObj) = t_dycHist;
    ObjqDycHist(iObj) = t_qDycHist;
end

== matlab function Noa_Nofusion_angle/TOS/Subsystem1/ACCOSM/HWA_Task100ms1/LostTargetCalc ==
  data: ObjValid input boolean size=15; ReID output uint8 size=1; ObjDx input single size=15; ObjDy input single size=15; DeltaDx input single size=1; DeltaDy input single size=1; P0IDK1 input uint8 size=1; P0VxK1 input single size=1; P0DxK1 input single size=1; P0DyK1 input single size=1; P0RangeK1 input; P0ArGK1 input; P0DycK1 input single size=1; P0VycK1 input single size=1; P0CutIn_bK1 input boolean size=1; tTargetLostK1 input single size=1; ReRange output single size=1; ReArG output single size=1; ReDx output single size=1; ReDy output single size=1; ReVx output single size=1; ReCutIn_b output boolean size=1; ReDyc output single size=1; ReVyc output single size=1; TargetLost_b output boolean size=1; Covered_b output boolean size=1; tTargetLost output single size=1
function [ReID,ReRange,ReArG,ReDx,ReDy,ReVx,ReCutIn_b,ReDyc,ReVyc,TargetLost_b,Covered_b,tTargetLost]...
    = LostTargetCalc(ObjValid,ObjDx,ObjDy,DeltaDx,DeltaDy,...
    P0IDK1,P0VxK1,P0DxK1,P0DyK1,P0RangeK1,P0ArGK1,P0DycK1,P0VycK1,P0CutIn_bK1,tTargetLostK1)
 
ReID = P0IDK1;
ReRange = single(255);
ReArG = single(0);
ReDx = single(255);
ReDy = single(0);
ReVx = single(0);
ReDyc = single(0);
ReVyc = single(0);
ReCutIn_b = false;
TargetLost_b = false;
tTargetLost = single(0);
Covered_b = false;
 
if (P0IDK1>0)&&(P0IDK1<100)    % k1 Exist Target
    if ObjValid(P0IDK1)==false
        ExistNearObj = false;
        P0DxPred = P0DxK1 + 0.1*P0VxK1;
        P0DyPred = P0DyK1;
        P0RangePred = P0RangeK1 + 0.1*P0VxK1; 
        for i=1:15
            if (ObjValid(i)==true)&&(ObjDx(i)<P0DxPred)
                Covered_b = CoveredCalc(P0DxPred,P0DyPred,ObjDx(i),ObjDy(i),single(2.1),single(-0.1));
                if Covered_b==true
                   break; 
                end
            end
            if (ObjValid(i)==1)&&(abs(ObjDx(i)-P0DxPred)<DeltaDx)&&(abs(ObjDy(i)-P0DyPred)<DeltaDy)
               ExistNearObj = true;
               ReID = uint8(i);
               ReDx = ObjDx(i);
            end
        end
        if (ExistNearObj==false)&&(Covered_b==false)
            TargetLost_b = true;
            tTargetLost = single(0.1);
            ReID = uint8(255);
            ReRange = P0RangePred;
            ReArG = P0ArGK1;
            ReDx = P0DxPred;
            ReDy = P0DyPred;
            ReVx = P0VxK1;
            ReCutIn_b = P0CutIn_bK1;
            ReVyc = P0VycK1;
            ReDyc = P0DycK1 + 0.1*P0VycK1;
        end
    end
else
    if P0IDK1>100   %  k1 Exist Target Re
        ExistNearObj = false;
        P0DxPred = P0DxK1 + 0.1*P0VxK1;
        P0DyPred = P0DyK1;
        P0RangePred = P0RangeK1 + 0.1*P0VxK1; 

        for i=1:15
            if (ObjValid(i)==1)&&(abs(ObjDx(i)-P0DxPred)<DeltaDx)&&(abs(ObjDy(i)-P0DyPred)<DeltaDy)
                ExistNearObj = true;
                ReID = uint8(i);
                ReDx = ObjDx(i);
                TargetLost_b = false;
                tTargetLost = single(0);
            end
        end
        if ExistNearObj==false
            TargetLost_b = true;
            tTargetLost = tTargetLostK1 + single(0.1);
            ReID = uint8(255);
            ReRange = P0RangePred;
            ReArG = P0ArGK1;
            ReDx = P0DxPred;
            ReDy = P0DyPred;
            ReVx = P0VxK1;
            ReCutIn_b = P0CutIn_bK1;
            ReVyc = P0VycK1;
            ReDyc = P0DycK1 + 0.1*P0VycK1;
        end
    end
end
end
 
function t_Covered_b = CoveredCalc(DxPred,DyPred,Dx,Dy,IFVDx,IFVDy)
y = (IFVDy - DyPred)*(Dx - DxPred)/(IFVDx - DxPred) + DyPred ;
Delta = single(0.8) + (Dx - IFVDx)/(DxPred - IFVDx);
if abs(Dy - y)<=Delta
    t_Covered_b = true;
else
    t_Covered_b = false;
end
end

== matlab function Noa_Nofusion_angle/TOS/Subsystem1/ACCOSM/HWA_Task100ms1/Lpb ==
  data: vRef input single size=1; alpSumSlideCurveness input single size=1; ObjValid input boolean size=15; ObjDyc input single size=15; ObjLpb output single size=15; ObjDycHist input single size=15; ObjqDycHist input single size=15; ObjLpbL output single size=15; ObjLpbR output single size=15; ObjVyc input single size=15; ObjYawAngle input single size=15; ObjDylaneEdgeRight input; ObjDyEdgeWidthRight input; ObjDylaneEdgeLeft input; ObjDyEdgeWidthLeft input
function [ObjLpb,ObjLpbL,ObjLpbR] = LpbCalc(vRef,alpSumSlideCurveness,...
    ObjValid,ObjDyc,ObjDycHist,ObjqDycHist,ObjVyc,ObjYawAngle,...
    ObjDylaneEdgeRight,ObjDyEdgeWidthRight,ObjDylaneEdgeLeft,ObjDyEdgeWidthLeft)

 [ObjLpb,ObjLpbL,ObjLpbR] = LpbCalc(vRef,alpSumSlideCurveness,...
    ObjValid,ObjDyc,ObjDycHist,ObjqDycHist,ObjVyc,ObjYawAngle,...
    ObjDylaneEdgeRight,ObjDyEdgeWidthRight,ObjDylaneEdgeLeft,ObjDyEdgeWidthLeft);
end

== matlab function Noa_Nofusion_angle/TOS/Subsystem1/ACCOSM/HWA_Task100ms1/Plaus ==
  data: dxMaxFollow input single size=1; ObjValid input boolean size=15; ObjDx input single size=15; ObjVx input single size=15; ObjPlaus output single size=15; ObjOnLeft input single size=15; ObjPlausLeft output single size=15; ObjPlausRight output single size=15; ObjOnRight input single size=15; ObjDycHist input single size=15; ObjqDycHist input single size=15; ObjLpb input single size=15; ObjLpbLeft input single size=15; ObjLpbRight input single size=15; ObjPlausK1 input single size=15; ObjPlausLeftK1 input single size=15; ObjPlausRightK1 input single size=15
function [ObjPlaus,ObjPlausLeft,ObjPlausRight] = ...
    PlausCalc(dxMaxFollow,ObjValid,ObjDx,ObjVx,ObjOnLeft,ObjOnRight,ObjDycHist,ObjqDycHist,...
    ObjLpb,ObjLpbLeft,ObjLpbRight,ObjPlausK1,ObjPlausLeftK1,ObjPlausRightK1)

[ObjPlaus,ObjPlausLeft,ObjPlausRight] = ...
    PlausCalc(dxMaxFollow,ObjValid,ObjDx,ObjVx,ObjOnLeft,ObjOnRight,ObjDycHist,ObjqDycHist,...
    ObjLpb,ObjLpbLeft,ObjLpbRight,ObjPlausK1,ObjPlausLeftK1,ObjPlausRightK1);
end

== matlab function Noa_Nofusion_angle/TOS/Subsystem1/ACCOSM/HWA_Task100ms1/Spw ==
  data: AlpSumSlideCurveness input single size=1; kapCourseErr input single size=1; ObjSpw output single size=15; ObjValid input boolean size=15; DycASI input single size=15; ObjDx input single size=15; ObjSpwLeft output single size=15; ObjSpwRight output single size=15; ObjOnLeft output; ObjOnRight output; ObjDyc input; ObjDycHist input; ObjqDycHist input; ObjDycASI output; ObjDyKapErr output
function [ObjSpw,ObjSpwLeft,ObjSpwRight,ObjOnLeft,ObjOnRight,ObjDycASI,ObjDyKapErr] = ...
    CalcSpw(AlpSumSlideCurveness,kapCourseErr,ObjValid,DycASI,ObjDx,ObjDyc,ObjDycHist,ObjqDycHist)
 
ObjSpw = single(zeros(15,1));
ObjSpwLeft = single(zeros(15,1));
ObjSpwRight = single(zeros(15,1));
ObjOnLeft = single(zeros(15,1));
ObjOnRight = single(zeros(15,1));
ObjDycASI = single(zeros(15,1));
ObjDyKapErr = single(zeros(15,1));
 
for i=1:15
    if ObjValid(i)
        t_dycASI = DycASI(i);
        t_kapErrMin = single(0.0002);
        t_kapErrCurvenessMax = single(0.0018);
        
        temp1 = min(AlpSumSlideCurveness,single(1));
        t_kapErrCurveness = t_kapErrCurvenessMax*temp1;
        t_kapErr = max(t_kapErrMin,max(kapCourseErr,t_kapErrCurveness));
        temp1 = min(ObjDx(i),single(80));
        t_DyKapErr = t_kapErr*temp1*temp1/2;
        ObjDyKapErr(i) = t_DyKapErr;
        
        %         t_dyHalfLane = 1.5;
        %         t_dy3halfLane = 5.25;
        
        if abs(t_dycASI)>=4.5
            t_spw = single(0);
            t_spwNeighbour = single(0);
        elseif abs(t_dycASI)>=3
            t_spw = single(0);
            t_dycToLane = abs(t_dycASI) - single(3);
            t_spwNeighbour = CalcSPW(t_dycToLane,single(3),t_DyKapErr);
        elseif abs(t_dycASI)>=1.5
            t_spw = single(0);
            t_spwNeighbour = CalcSPW(single(0),single(3),t_DyKapErr);
        else
            t_spwNeighbour = single(0);
            t_spw = CalcSPW(single(0),single(3),t_DyKapErr);
        end
        if t_dycASI>=0
            t_spwRight = single(0);
            t_spwLeft = t_spwNeighbour;
        else
            t_spwLeft = single(0);
            t_spwRight = t_spwNeighbour;
        end
        ObjSpw(i) = t_spw;
        ObjSpwLeft(i) = t_spwLeft;
        ObjSpwRight(i) = t_spwRight;
        % -------------------------------------------------------------------------
        
        temp1 = 0.5*ObjqDycHist(i);
        t_dycASI = ObjDyc(i)*(1-temp1) + ObjDycHist(i)*temp1;
        temp2 = single(1.5) + t_DyKapErr;
        temp3 = single(3) + t_DyKapErr;
        ObjDycASI(i) = t_dycASI;
        
        if t_dycASI>=0
            temp1 = max(single(1.5),min(temp3,t_dycASI)) - single(1.5);
            ObjOnLeft(i) = min(single(1),temp1/temp2);
        else
            temp1 = max(min(single(-1.5),t_dycASI),-temp3);
            temp1 = -temp1 - single(1.5);
            ObjOnRight(i) = min(single(1),temp1/temp2);
        end
    end
end
end
 
function t_spw = CalcSPW(absDyc,dyLaneWidth,dyKapErr)
temp3 = dyLaneWidth/2;
temp1 = temp3 - dyKapErr;
temp2 = temp3 + dyKapErr;
temp2 = min(temp2,dyLaneWidth);
 
if absDyc<=temp1
    t_spw = single(1);
elseif absDyc>=temp2
    t_spw = single(0);
else
    temp3 = temp2 - absDyc;
    temp4 = 2*dyKapErr;
    t_spw = temp3/temp4;
end
end

== matlab function Noa_Nofusion_angle/TOS/Subsystem1/ACCOSM/HWA_Task100ms1/Std ==
  data: u input; y output
function y = fcn(u)

y = std(u);

== matlab function Noa_Nofusion_angle/TOS/Subsystem1/ACCOSM/HWA_Task100ms1/TargetBrake ==
  data: ID input uint8; VxG input; VyG input; TargetBrake_b output boolean; TargetVxG output; BrakeLightIndic input uint8 size=15; TargetVyG output
function [TargetBrake_b,TargetVxG,TargetVyG] = fcn(ID,VxG,VyG,BrakeLightIndic)
%#codegen
TargetBrake_b = false;
TargetVxG = single(0);
TargetVyG = single(0);

if (ID>0)&&(ID<100)
    if BrakeLightIndic(ID)==2
        TargetBrake_b = true;
    end
    TargetVxG = VxG(ID);
    TargetVyG = VyG(ID);
end
